simulink model "BS_NN"  (R2025a)
settings: Solver=ode45  StartTime=0.0  StopTime=50  RelTol=1e-3
libraries: eeGeneralControl x15, uavutilslib x1
settings Model: SimulationMode=accelerator  Creator=vinh1  LastModifiedBy=vinh1
settings DebuggingCC: AlgebraicLoopMsg=none

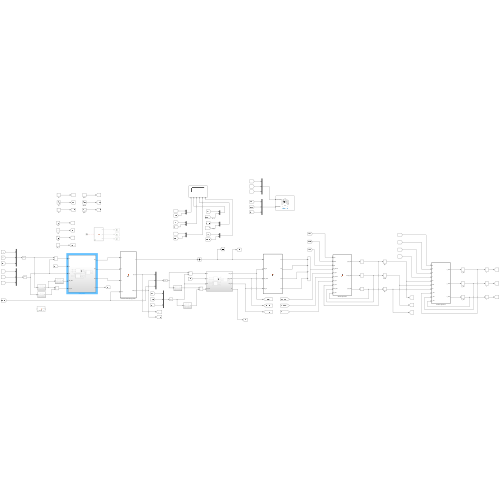
[thumbnail: Simulink's stored preview of the top-level diagram]
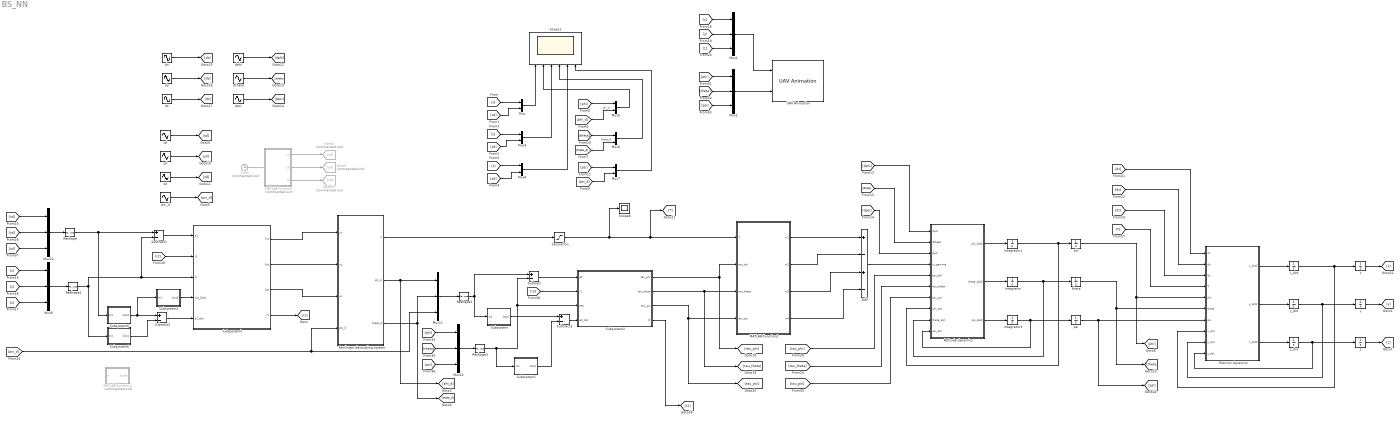
== system BS_NN ==
  Add : Sum  Inputs=+-+-
  Attitude dynamics : MATLAB Function  TreatAsAtomicUnit=on
  Clock : Clock  Commented=on
      settings: Decimation=50
  Goto2 : Goto  Commented=on  GotoTag=xd
  Goto25 : Goto  Commented=on  GotoTag=zd
  Goto6 : Goto  Commented=on  GotoTag=yd
  Integrator : Integrator
  Integrator1 : Integrator
  Integrator3 : Integrator
  MATLAB Function : MATLAB Function  Commented=on  TreatAsAtomicUnit=on
  MATLAB Function1 : MATLAB Function  Commented=on  TreatAsAtomicUnit=on
  MATLAB Function2 : MATLAB Function  TreatAsAtomicUnit=on
  Mux{,3..7} (6 alike) : Mux  Inputs=2
  Mux{1..2,9..12} (6 alike) : Mux  Inputs=3
  Nonlinear decoupling system : MATLAB Function  TreatAsAtomicUnit=on
  Position dynamics : MATLAB Function  TreatAsAtomicUnit=on
  Reshape{,2..4} (4 alike) : Reshape  OutputDimensionality=Customize  OutputDimensions=[3,1]
  Saturation : Saturate  UpperLimit=130  LowerLimit=0
  Scope1 : Scope  NumInputPorts=6
      settings: ActiveDisplayString=6  ActiveDisplayYMinimum=-0.00010356739375247082  ActiveDisplayYMaximum=0.00093210654377223767
  Scope6 : Scope
      settings: ActiveDisplayYMinimum=9.3887609139201285  ActiveDisplayYMaximum=11.61040929343401  DataLoggingVariableName=ScopeData6
  Subsystem : Subsystem
  Subsystem1 : Subsystem
  Subsystem2 : Subsystem
  Subsystem3 : Subsystem
  Subsystem4 : Subsystem
  Subsystem5 : Subsystem
  Subsystem6 : Subsystem
  Subtract{,1..3} (4 alike) : Sum  Inputs=+-
  UAV Animation : uavutilslib/UAV Animation  NumUAV=1  DynamicUAVConfig=off  UAVType=Multirotor  UAVSize=1  UAVColor=[1 0 0]  UAVTrajectoryAlpha=1  InertialZDirection=Up  RotationFormat=Euler ZYX  DrawMarkers=off  SampleTime=-1
  dphi : Sin  Amplitude=0.2  Frequency=2  SampleTime=0
  dpsi : Sin  Amplitude=0.1  SampleTime=0
  dtheta : Sin  Amplitude=0.2  Frequency=2  SampleTime=0
  dx : Sin  Amplitude=0.3  SampleTime=0
  dy : Sin  Amplitude=0.3  SampleTime=0
  dz : Sin  Amplitude=0.1  Frequency=0.5  Phase=pi/2  SampleTime=0
  phi : Integrator
  psi : Integrator
  psi_d : Sin  Amplitude=0  Frequency=pi/10  Phase=pi/2  SampleTime=0
  theta : Integrator  LimitOutput=on  UpperSaturationLimit=85*pi/180  LowerSaturationLimit=-85*pi/180
  x : Integrator
  x_dot : Integrator
  xd : Sin  Amplitude=0.5  Frequency=pi/10  Phase=pi/2  SampleTime=0
  y : Integrator
  y_dot : Integrator
  yd : Sin  Amplitude=0.5  Frequency=pi/10  SampleTime=0
  z : Integrator  InitialCondition=2  LimitOutput=on  UpperSaturationLimit=100  LowerSaturationLimit=0
  z_dot : Integrator
  zd : Sin  Amplitude=0.5  Bias=2  Frequency=pi/10  Phase=3*pi/2  SampleTime=0
  wires:
  z_dot/1 -> z/1, Position dynamics/10(z_dot)
  z/1 -> [z]
  MATLAB Function2/2(w2) -> Add/2
  Mux2/1 -> UAV Animation/1
  [T] -> Position dynamics/4(T)
  [phi_d] -> Mux5/2  "phi_d"
  Nonlinear decoupling system/3(theta_d) -> Mux11/2, [theta_d]
  theta/1 -> [theta], Position dynamics/6(theta)
  [dpsi] -> Attitude dynamics/3(dpsi)
  [y] -> Mux3/1
  Mux4/1 -> Scope1/5
  [theta_d] -> Mux6/2  "theta_d"
  [psi] -> Mux7/1
  dz/1 -> [dz]
  [tau_phi] -> Attitude dynamics/5(tau_phi)
  phi/1 -> [phi], Position dynamics/5(phi)
  [psi_d] -> Mux7/2
  Subsystem3/1(fxd) -> Nonlinear decoupling system/1(ux)
  Subsystem2/3(tau_psi) -> [tau_psi], MATLAB Function2/4(tau_psi)
  dtheta/1 -> [dtheta]
  dx/1 -> [dx]
  [phi] -> Mux5/1
  Add/1 -> Attitude dynamics/4(w_gamma)
  Mux6/1 -> Scope1/4
  Saturation/1 -> Scope6/1, [T], MATLAB Function2/1(T)
  [tau_theta] -> Attitude dynamics/6(tau_theta)
  [yd] -> Mux3/2
  Position dynamics/3(z_dot2) -> z_dot/1
  [theta] -> Mux6/1
  Subsystem3/3(fzd) -> Nonlinear decoupling system/3(uz)
  y_dot/1 -> y/1, Position dynamics/9(y_dot)
  dy/1 -> [dy]
  [psi_d] -> Mux11/3, Nonlinear decoupling system/4(psi_d)
  [dz] -> Position dynamics/3(dz)
  Mux3/1 -> Scope1/3
  [dx] -> Position dynamics/1(dx)
  [y] -> Mux2/2
  Position dynamics/1(x_dot2) -> x_dot/1
  MATLAB Function2/4(w4) -> Add/4
  [dtheta] -> Attitude dynamics/2(dtheta)
  [x] -> Mux/1
  dpsi/1 -> [dpsi]
  [z] -> Mux4/1
  [z] -> Mux2/3
  Nonlinear decoupling system/1(T) -> Saturation/1
  psi_d/1 -> [psi_d]
  [x] -> Mux2/1
  Mux/1 -> Scope1/1
  [zd] -> Mux4/2
  Mux7/1 -> Scope1/6
  [xd] -> Mux/2
  y/1 -> [y]
  MATLAB Function/3(zd) -> Goto25/1
  Mux5/1 -> Scope1/2
  MATLAB Function/2(yd) -> Goto6/1
  yd/1 -> [yd]
  x_dot/1 -> x/1, Position dynamics/8(x_dot)
  zd/1 -> [zd]
  x/1 -> [x]
  Subsystem2/1(tau_phi) -> [tau_phi], MATLAB Function2/2(tau_phi)
  dphi/1 -> [dphi]
  xd/1 -> [xd]
  [theta] -> Mux1/2
  MATLAB Function2/1(w1) -> Add/1
  [dy] -> Position dynamics/2(dy)
  MATLAB Function/1(xd) -> Goto2/1
  psi/1 -> [psi], Position dynamics/7(psi)
  [dphi] -> Attitude dynamics/1(dphi)
  [phi] -> Mux1/1
  Mux1/1 -> UAV Animation/2
  [psi] -> Mux1/3
  Position dynamics/2(y_dot2) -> y_dot/1
  [tau_psi] -> Attitude dynamics/7(tau_psi)
  Subsystem3/2(fyd) -> Nonlinear decoupling system/2(uy)
  Clock/1 -> ?
  MATLAB Function2/3(w3) -> Add/3
  Subsystem2/2(tau_theta) -> [tau_theta], MATLAB Function2/3(tau_theta)
  Nonlinear decoupling system/2(phi_d) -> Mux11/1, [phi_d]
  Subtract/1 -> Subsystem2/1(e2)
  [phi] -> Mux12/1
  [theta] -> Mux12/2
  [psi] -> Mux12/3
  [xd] -> Mux10/1
  [yd] -> Mux10/2
  [zd] -> Mux10/3
  [x] -> Mux9/1
  [y] -> Mux9/2
  [z] -> Mux9/3
  Subtract1/1 -> Subsystem3/1(e1)
  [r1] -> Subsystem2/2(r1)
  Subsystem3/4(r1) -> [r1]
  Subsystem2/4(r2) -> [r2]
  [r2] -> Subsystem3/2(r2)
  Reshape4/1 -> Subsystem3/3(Xi), Subtract1/2, Subsystem6/1(In1)
  Reshape/1 -> Subsystem5/1(In1), Subtract1/1
  Mux11/1 -> Reshape2/1
  Reshape2/1 -> Subsystem/1(In1), Subtract/1
  Mux12/1 -> Reshape3/1
  Attitude dynamics/1(phi_dot2) -> Integrator1/1
  Attitude dynamics/3(psi_dot2) -> Integrator3/1
  Attitude dynamics/2(theta_dot2) -> Integrator/1
  Subsystem4/1(Out1) -> Subsystem3/4(Xid_2dot)
  Integrator/1 -> Attitude dynamics/9(theta_dot), theta/1
  Integrator1/1 -> phi/1, Attitude dynamics/8(phi_dot)
  Integrator3/1 -> Attitude dynamics/10(psi_dot), psi/1
  Reshape3/1 -> Subsystem1/1(In1), Subtract/2, Subsystem2/3(eta)
  Subtract3/1 -> Subsystem2/4(e2_dot)
  Subsystem1/1(Out1) -> Subtract3/2
  Subsystem5/1(Out1) -> Subsystem4/1(In1), Subtract2/1
  Subsystem6/1(Out1) -> Subtract2/2
  Subtract2/1 -> Subsystem3/5(e1_dot)
  Mux10/1 -> Reshape/1
  Mux9/1 -> Reshape4/1
  Subsystem/1(Out1) -> Subtract3/1

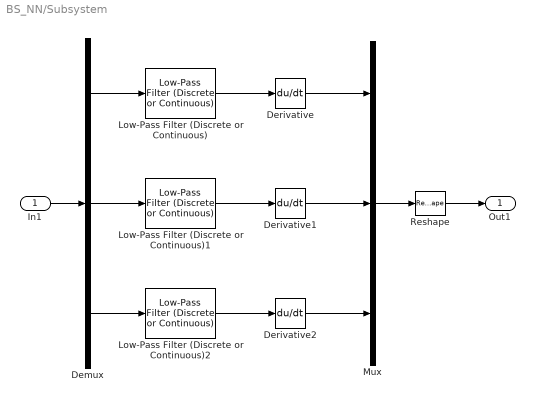
== system BS_NN/Subsystem ==
  In1 : Inport
  Demux : Demux  Outputs=3
  Derivative : Derivative
  Derivative1 : Derivative
  Derivative2 : Derivative
  Low-Pass Filter (Discrete or Continuous) : eeGeneralControl/Low-Pass Filter (Discrete or Continuous)  K=1  T=0.01  B=inf  A=-inf  init_option=Inherited from block input  x0=0  Ts=0
  Low-Pass Filter (Discrete or Continuous)1 : eeGeneralControl/Low-Pass Filter (Discrete or Continuous)  K=1  T=0.01  B=inf  A=-inf  init_option=Inherited from block input  x0=0  Ts=0
  Low-Pass Filter (Discrete or Continuous)2 : eeGeneralControl/Low-Pass Filter (Discrete or Continuous)  K=1  T=0.01  B=inf  A=-inf  init_option=Inherited from block input  x0=0  Ts=0
  Mux : Mux  Inputs=3
  Reshape : Reshape  OutputDimensionality=Column vector (2-D)
  Out1 : Outport
  wires:
  In1/1 -> Demux/1
  Demux/1 -> Low-Pass Filter (Discrete or Continuous)/1
  Demux/2 -> Low-Pass Filter (Discrete or Continuous)1/1
  Demux/3 -> Low-Pass Filter (Discrete or Continuous)2/1
  Low-Pass Filter (Discrete or Continuous)/1 -> Derivative/1
  Low-Pass Filter (Discrete or Continuous)1/1 -> Derivative1/1
  Low-Pass Filter (Discrete or Continuous)2/1 -> Derivative2/1
  Derivative2/1 -> Mux/3
  Derivative/1 -> Mux/1
  Derivative1/1 -> Mux/2
  Mux/1 -> Reshape/1
  Reshape/1 -> Out1/1

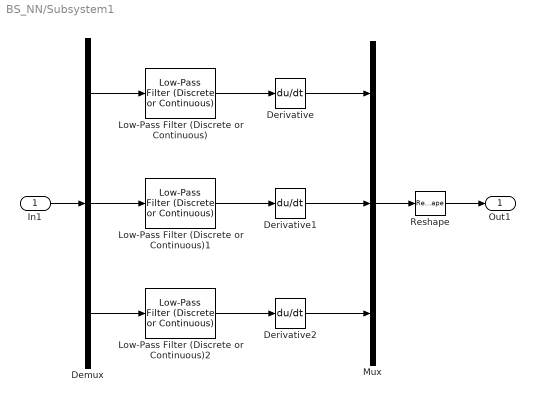
== system BS_NN/Subsystem1 ==
  In1 : Inport
  Demux : Demux  Outputs=3
  Derivative : Derivative
  Derivative1 : Derivative
  Derivative2 : Derivative
  Low-Pass Filter (Discrete or Continuous) : eeGeneralControl/Low-Pass Filter (Discrete or Continuous)  K=1  T=0.01  B=inf  A=-inf  init_option=Inherited from block input  x0=0  Ts=0
  Low-Pass Filter (Discrete or Continuous)1 : eeGeneralControl/Low-Pass Filter (Discrete or Continuous)  K=1  T=0.01  B=inf  A=-inf  init_option=Inherited from block input  x0=0  Ts=0
  Low-Pass Filter (Discrete or Continuous)2 : eeGeneralControl/Low-Pass Filter (Discrete or Continuous)  K=1  T=0.01  B=inf  A=-inf  init_option=Inherited from block input  x0=0  Ts=0
  Mux : Mux  Inputs=3
  Reshape : Reshape  OutputDimensionality=Column vector (2-D)
  Out1 : Outport
  wires:
  Reshape/1 -> Out1/1
  Mux/1 -> Reshape/1
  Derivative1/1 -> Mux/2
  Derivative/1 -> Mux/1
  Derivative2/1 -> Mux/3
  Low-Pass Filter (Discrete or Continuous)2/1 -> Derivative2/1
  Low-Pass Filter (Discrete or Continuous)1/1 -> Derivative1/1
  Low-Pass Filter (Discrete or Continuous)/1 -> Derivative/1
  Demux/3 -> Low-Pass Filter (Discrete or Continuous)2/1
  Demux/2 -> Low-Pass Filter (Discrete or Continuous)1/1
  Demux/1 -> Low-Pass Filter (Discrete or Continuous)/1
  In1/1 -> Demux/1

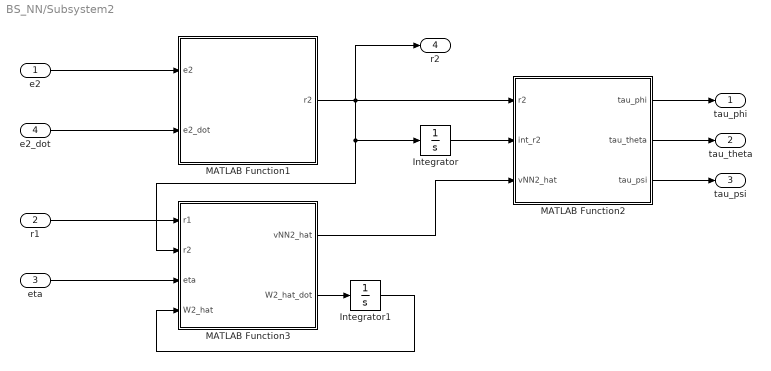
== system BS_NN/Subsystem2 ==
  e2 : Inport
  r1 : Inport  Port=2
  eta : Inport  Port=3
  e2_dot : Inport  Port=4
  Integrator : Integrator  InitialCondition=zeros(3,1)
  Integrator1 : Integrator  InitialCondition=zeros(9,3)
  MATLAB Function1 : MATLAB Function  TreatAsAtomicUnit=on
  MATLAB Function2 : MATLAB Function  TreatAsAtomicUnit=on
  MATLAB Function3 : MATLAB Function  TreatAsAtomicUnit=on
  tau_phi : Outport
  tau_theta : Outport  Port=2
  tau_psi : Outport  Port=3
  r2 : Outport  Port=4
  wires:
  MATLAB Function2/3(tau_psi) -> tau_psi/1
  MATLAB Function2/2(tau_theta) -> tau_theta/1
  MATLAB Function2/1(tau_phi) -> tau_phi/1
  Integrator1/1 -> MATLAB Function3/4(W2_hat)
  MATLAB Function3/2(W2_hat_dot) -> Integrator1/1
  eta/1 -> MATLAB Function3/3(eta)
  MATLAB Function3/1(vNN2_hat) -> MATLAB Function2/3(vNN2_hat)
  Integrator/1 -> MATLAB Function2/2(int_r2)
  MATLAB Function1/1(r2) -> r2/1, MATLAB Function2/1(r2), Integrator/1, MATLAB Function3/2(r2)
  e2/1 -> MATLAB Function1/1(e2)
  r1/1 -> MATLAB Function3/1(r1)
  e2_dot/1 -> MATLAB Function1/2(e2_dot)

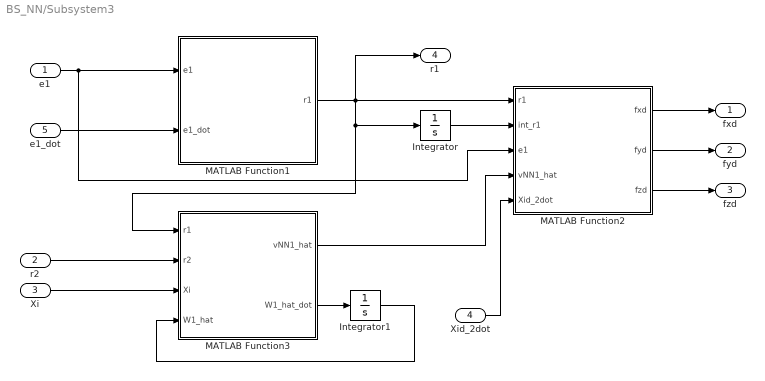
== system BS_NN/Subsystem3 ==
  e1 : Inport
  r2 : Inport  Port=2
  Xi : Inport  Port=3
  Xid_2dot : Inport  Port=4
  e1_dot : Inport  Port=5
  Integrator : Integrator  InitialCondition=zeros(3,1)
  Integrator1 : Integrator  InitialCondition=zeros(9,3)
  MATLAB Function1 : MATLAB Function  TreatAsAtomicUnit=on
  MATLAB Function2 : MATLAB Function  TreatAsAtomicUnit=on
  MATLAB Function3 : MATLAB Function  TreatAsAtomicUnit=on
  fxd : Outport
  fyd : Outport  Port=2
  fzd : Outport  Port=3
  r1 : Outport  Port=4
  wires:
  MATLAB Function2/3(fzd) -> fzd/1
  MATLAB Function2/2(fyd) -> fyd/1
  MATLAB Function2/1(fxd) -> fxd/1
  Integrator1/1 -> MATLAB Function3/4(W1_hat)
  MATLAB Function3/2(W1_hat_dot) -> Integrator1/1
  Xi/1 -> MATLAB Function3/3(Xi)
  MATLAB Function3/1(vNN1_hat) -> MATLAB Function2/4(vNN1_hat)
  Integrator/1 -> MATLAB Function2/2(int_r1)
  MATLAB Function1/1(r1) -> MATLAB Function3/1(r1), Integrator/1, MATLAB Function2/1(r1), r1/1
  e1/1 -> MATLAB Function2/3(e1), MATLAB Function1/1(e1)
  r2/1 -> MATLAB Function3/2(r2)
  Xid_2dot/1 -> MATLAB Function2/5(Xid_2dot)
  e1_dot/1 -> MATLAB Function1/2(e1_dot)

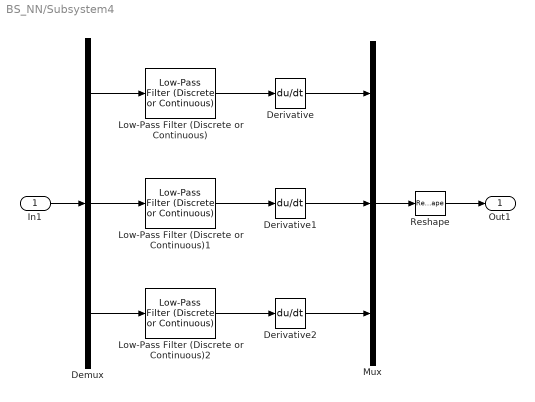
== system BS_NN/Subsystem4 ==
  In1 : Inport
  Demux : Demux  Outputs=3
  Derivative : Derivative
  Derivative1 : Derivative
  Derivative2 : Derivative
  Low-Pass Filter (Discrete or Continuous) : eeGeneralControl/Low-Pass Filter (Discrete or Continuous)  K=1  T=0.01  B=inf  A=-inf  init_option=Inherited from block input  x0=0  Ts=0
  Low-Pass Filter (Discrete or Continuous)1 : eeGeneralControl/Low-Pass Filter (Discrete or Continuous)  K=1  T=0.01  B=inf  A=-inf  init_option=Inherited from block input  x0=0  Ts=0
  Low-Pass Filter (Discrete or Continuous)2 : eeGeneralControl/Low-Pass Filter (Discrete or Continuous)  K=1  T=0.01  B=inf  A=-inf  init_option=Inherited from block input  x0=0  Ts=0
  Mux : Mux  Inputs=3
  Reshape : Reshape  OutputDimensionality=Column vector (2-D)
  Out1 : Outport
  wires:
  Reshape/1 -> Out1/1
  Mux/1 -> Reshape/1
  Derivative1/1 -> Mux/2
  Derivative/1 -> Mux/1
  Derivative2/1 -> Mux/3
  Low-Pass Filter (Discrete or Continuous)2/1 -> Derivative2/1
  Low-Pass Filter (Discrete or Continuous)1/1 -> Derivative1/1
  Low-Pass Filter (Discrete or Continuous)/1 -> Derivative/1
  Demux/3 -> Low-Pass Filter (Discrete or Continuous)2/1
  Demux/2 -> Low-Pass Filter (Discrete or Continuous)1/1
  Demux/1 -> Low-Pass Filter (Discrete or Continuous)/1
  In1/1 -> Demux/1

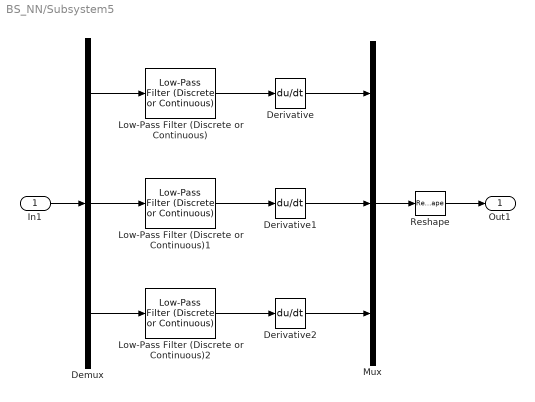
== system BS_NN/Subsystem5 ==
  In1 : Inport
  Demux : Demux  Outputs=3
  Derivative : Derivative
  Derivative1 : Derivative
  Derivative2 : Derivative
  Low-Pass Filter (Discrete or Continuous) : eeGeneralControl/Low-Pass Filter (Discrete or Continuous)  K=1  T=0.01  B=inf  A=-inf  init_option=Inherited from block input  x0=0  Ts=0
  Low-Pass Filter (Discrete or Continuous)1 : eeGeneralControl/Low-Pass Filter (Discrete or Continuous)  K=1  T=0.01  B=inf  A=-inf  init_option=Inherited from block input  x0=0  Ts=0
  Low-Pass Filter (Discrete or Continuous)2 : eeGeneralControl/Low-Pass Filter (Discrete or Continuous)  K=1  T=0.01  B=inf  A=-inf  init_option=Inherited from block input  x0=0  Ts=0
  Mux : Mux  Inputs=3
  Reshape : Reshape  OutputDimensionality=Column vector (2-D)
  Out1 : Outport
  wires:
  Reshape/1 -> Out1/1
  Mux/1 -> Reshape/1
  Derivative1/1 -> Mux/2
  Derivative/1 -> Mux/1
  Derivative2/1 -> Mux/3
  Low-Pass Filter (Discrete or Continuous)2/1 -> Derivative2/1
  Low-Pass Filter (Discrete or Continuous)1/1 -> Derivative1/1
  Low-Pass Filter (Discrete or Continuous)/1 -> Derivative/1
  Demux/3 -> Low-Pass Filter (Discrete or Continuous)2/1
  Demux/2 -> Low-Pass Filter (Discrete or Continuous)1/1
  Demux/1 -> Low-Pass Filter (Discrete or Continuous)/1
  In1/1 -> Demux/1

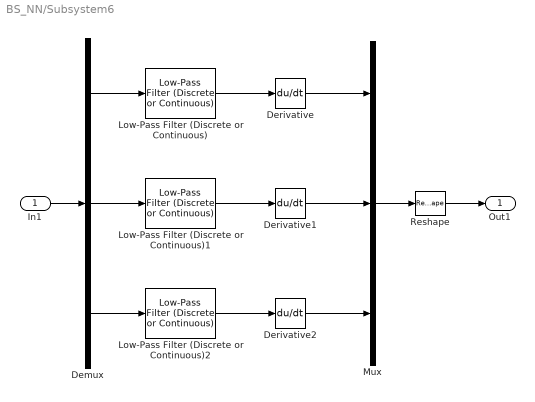
== system BS_NN/Subsystem6 ==
  In1 : Inport
  Demux : Demux  Outputs=3
  Derivative : Derivative
  Derivative1 : Derivative
  Derivative2 : Derivative
  Low-Pass Filter (Discrete or Continuous) : eeGeneralControl/Low-Pass Filter (Discrete or Continuous)  K=1  T=0.01  B=inf  A=-inf  init_option=Inherited from block input  x0=0  Ts=0
  Low-Pass Filter (Discrete or Continuous)1 : eeGeneralControl/Low-Pass Filter (Discrete or Continuous)  K=1  T=0.01  B=inf  A=-inf  init_option=Inherited from block input  x0=0  Ts=0
  Low-Pass Filter (Discrete or Continuous)2 : eeGeneralControl/Low-Pass Filter (Discrete or Continuous)  K=1  T=0.01  B=inf  A=-inf  init_option=Inherited from block input  x0=0  Ts=0
  Mux : Mux  Inputs=3
  Reshape : Reshape  OutputDimensionality=Column vector (2-D)
  Out1 : Outport
  wires:
  In1/1 -> Demux/1
  Demux/1 -> Low-Pass Filter (Discrete or Continuous)/1
  Demux/2 -> Low-Pass Filter (Discrete or Continuous)1/1
  Demux/3 -> Low-Pass Filter (Discrete or Continuous)2/1
  Low-Pass Filter (Discrete or Continuous)/1 -> Derivative/1
  Low-Pass Filter (Discrete or Continuous)1/1 -> Derivative1/1
  Low-Pass Filter (Discrete or Continuous)2/1 -> Derivative2/1
  Derivative2/1 -> Mux/3
  Derivative/1 -> Mux/1
  Derivative1/1 -> Mux/2
  Mux/1 -> Reshape/1
  Reshape/1 -> Out1/1

== matlab function BS_NN/MATLAB Function ==
  data: xd output; yd output; zd output
function [xd, yd, zd] = fcn()

%w0 = pi/10;
%xd = 2*sin(w0*t)*cos(w0*t/2);

%yd = 2*sin(w0*t)*sin(w0*t/2);

%zd = 2 -sin(w0*t)*(cos(w0*t/2) + sin(w0*t/2));
xd = 5;
yd = 10;
zd = 5;

== matlab function BS_NN/Subsystem2/MATLAB Function2 ==
  data: r2 input size=[3 1]; tau_phi output; int_r2 input size=[3 1]; tau_theta output; tau_psi output; vNN2_hat input size=[3 1]
function [tau_phi, tau_theta, tau_psi] = fcn(r2, int_r2, vNN2_hat)

Kr2 = [0.6; 0.6; 0.4];
Ki2 = [0.01; 0.01; 0.0148];

tau = vNN2_hat + Kr2.*r2 + Ki2.*int_r2;

tau_phi = tau(1);
tau_theta = tau(2);
tau_psi = tau(3);

== matlab function BS_NN/Subsystem2/MATLAB Function3 ==
  data: r1 input size=[3 1]; r2 input size=[3 1]; vNN2_hat output size=[3 1]; eta input size=[3 1]; W2_hat_dot output size=[9 3]; W2_hat input size=[9 3]
function [vNN2_hat, W2_hat_dot] = NN2(r1, r2, eta, W2_hat)

Chi2 = [r1; r2; eta];
r = [r1; r2];

F2 = 0.001;
k = 3;

nuy2 = tanh(Chi2);
vNN2_hat = W2_hat'*nuy2;

W2_hat_dot = F2*nuy2*r2' - k*norm(r)*F2*W2_hat;

== matlab function BS_NN/Subsystem3/MATLAB Function1 ==
  settings: updateMethod=DISCRETE
  data: e1 input size=[3 1]; r1 output size=[3 1]; e1_dot input
function r1 = fcn(e1,e1_dot)

Lambda1 = diag([2 2 2]);

r1 = e1_dot + Lambda1*e1;

== matlab function BS_NN/Subsystem3/MATLAB Function2 ==
  data: r1 input size=[3 1]; fxd output; int_r1 input size=[3 1]; e1 input size=[3 1]; fyd output; fzd output; vNN1_hat input size=[3 1]; Xid_2dot input size=[3 1]
function [fxd, fyd, fzd] = fcn(r1, int_r1, e1, vNN1_hat, Xid_2dot)

Kr1 = [3; 3; 3];
Ki1 = [0.5; 0.5; 0.5];

Lambda1 = diag([2 2 2]);

m = 1.121;
g = 9.81;
m_g = [0; 0; -m*g];

Fd_hat = m*Xid_2dot - m*Lambda1^2*e1 - m_g + vNN1_hat + Kr1.*r1 + Ki1.*int_r1;

fxd = Fd_hat(1);
fyd = Fd_hat(2);
fzd = Fd_hat(3);

== matlab function BS_NN/Subsystem3/MATLAB Function3 ==
  data: r1 input size=[3 1]; r2 input size=[3 1]; vNN1_hat output size=[3 1]; Xi input size=[3 1]; W1_hat_dot output size=[9 3]; W1_hat input size=[9 3]
function [vNN1_hat, W1_hat_dot] = NN1(r1, r2, Xi, W1_hat)

Chi1 = [r1; r2; Xi];
r = [r1; r2];

F1 = 4;
k = 5;

nuy1 = tanh(Chi1);
vNN1_hat = W1_hat'*nuy1;

W1_hat_dot = F1*nuy1*r1' - k*norm(r)*F1*W1_hat;

== matlab function BS_NN/Attitude dynamics ==
  data: dphi input; dtheta input; dpsi input; w_gamma input; phi_dot2 output; tau_phi input; tau_theta input; tau_psi input; theta_dot2 output; psi_dot2 output; phi_dot input; theta_dot input; psi_dot input
function [phi_dot2, theta_dot2, psi_dot2] = fcn(dphi, dtheta, dpsi, w_gamma, tau_phi, tau_theta, tau_psi, phi_dot, theta_dot, psi_dot)

Ixx = 0.01 ;
Iyy = 0.01 ; 
Izz = 0.0148 ;
Ir = 2.83e-5 ;

phi_dot2 = theta_dot*psi_dot*(Iyy - Izz)/Ixx - theta_dot*w_gamma*Ir/Ixx + tau_phi/Ixx + dphi;

theta_dot2 = phi_dot*psi_dot*(Izz - Ixx)/Iyy + phi_dot*w_gamma*Ir/Iyy + tau_theta/Iyy + dtheta;

psi_dot2 = phi_dot*theta_dot*(Ixx - Iyy)/Izz + tau_psi/Izz + dpsi;

end

== matlab function BS_NN/Nonlinear decoupling system ==
  data: ux input; T output; uy input; uz input; psi_d input; phi_d output; theta_d output
function [T, phi_d, theta_d] = fcn(ux, uy, uz, psi_d)

m = 1.121 ;
g = 9.81 ;

T = sqrt( (ux)^2 + (uy)^2 + (uz)^2);

phi_d = asin((ux*sin(psi_d) - uy*cos(psi_d)) / (T));

theta_d = atan((ux*cos(psi_d) + uy*sin(psi_d)) / (uz));

== matlab function BS_NN/MATLAB Function2 ==
  data: T input; w1 output; tau_phi input; tau_theta input; tau_psi input; w2 output; w3 output; w4 output
function [w1, w2, w3, w4] = fcn(T, tau_phi, tau_theta, tau_psi)

k = 2.98e-5 ;
l = 0.25 ;
b = 3.23e-7 ;

w1 = sqrt(max(0,(T/(4*k)) - (tau_theta/(2*k*l)) - (tau_psi/(4*b))));

w2 = sqrt(max(0,(T/(4*k)) - (tau_phi /(2*k*l)) + (tau_psi/(4*b))));

w3 = sqrt(max(0,(T/(4*k)) + (tau_theta/(2*k*l)) - (tau_psi/(4*b))));

w4 = sqrt(max(0,(T/(4*k)) + (tau_phi /(2*k*l)) + (tau_psi/(4*b))));

end

== matlab function BS_NN/Position dynamics ==
  data: dx input; dy input; dz input; T input; phi input; x_dot2 output; theta input; psi input; x_dot input; y_dot2 output; z_dot2 output; y_dot input; z_dot input
function [x_dot2, y_dot2, z_dot2] = fcn(dx, dy, dz, T, phi, theta, psi, x_dot, y_dot, z_dot)

Ax = 5.56e-4 ;
Ay = 5.56e-4 ;
Az = 6.35e-4 ;

m = 1.121 ;
g = 9.81 ;

x_dot2 = (T/m)*(cos(phi)*sin(theta)*cos(psi) + sin(phi)*sin(psi)) - (Ax/m)*x_dot + dx;

y_dot2 = (T/m)*(cos(phi)*sin(theta)*sin(psi) - sin(phi)*cos(psi)) - (Ay/m)*y_dot + dy;

z_dot2 = (T/m)*cos(phi)*cos(theta) - g - (Az/m)*z_dot + dz;

end

== matlab function BS_NN/MATLAB Function1 ==
  data: e input; e_dot output
function e_dot = Derivative(e)

Ts = 0.005;

persistent e_prev e_prev1
if isempty(e_prev)
    e_prev  = zeros(3,1);
    e_prev1 = zeros(3,1);
end

e_dot = (e_prev1 - e_prev)/Ts;

e_prev1 = e_prev;
e_prev = e;

== matlab function BS_NN/Subsystem2/MATLAB Function1 ==
  data: e2 input size=[3 1]; r2 output size=[3 1]; e2_dot input size=[3 1]
function r2 = fcn(e2, e2_dot)

Lambda2 = diag([4 4 4]);

r2 = e2_dot + Lambda2*e2;
